simulink model "propagator"  (R2019b)
settings: Solver=VariableStepAuto  StartTime=0.0  StopTime=10.0  RelTol=1e-3
model workspace (MAT data in the model file):
  X0 = 1
  mi = 1
settings Model: Creator=antoniogenova  LastModifiedBy=antoniogenova

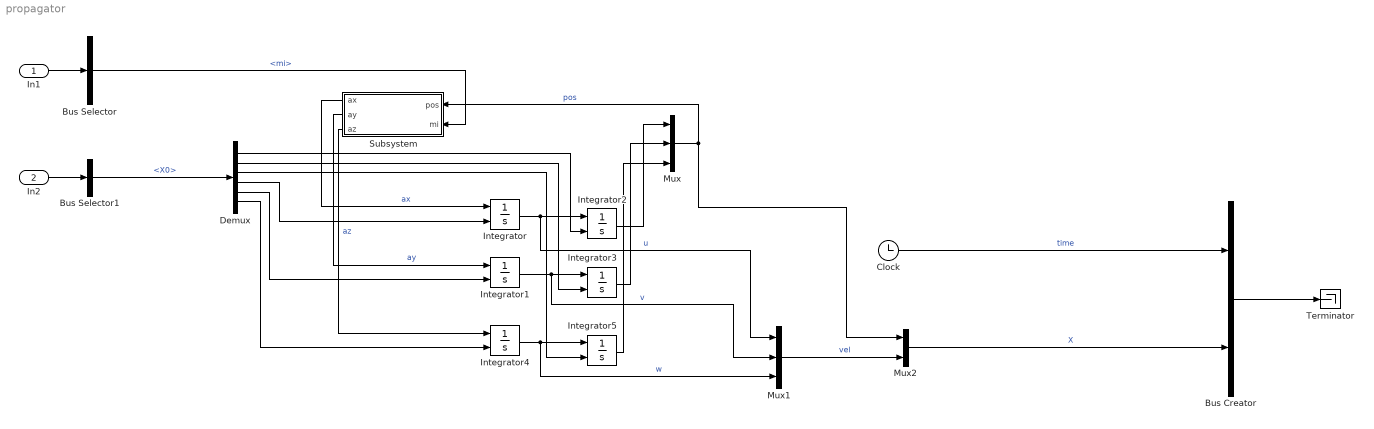
== system propagator ==
  In1 : Inport  OutDataTypeStr=Bus: ParBody_Bus
  In2 : Inport  Port=2  OutDataTypeStr=Bus: ParEphemerides_Bus
  Bus Creator : BusCreator  Inputs=2
  Bus Selector : BusSelector  OutputSignals=mi
  Bus Selector1 : BusSelector  OutputSignals=X0
  Clock : Clock
  Demux : Demux  Outputs=6
  Integrator{,1..5} (6 alike) : Integrator  InitialConditionSource=external  ContinuousStateAttributes="\"\""
  Mux : Mux  Inputs=3
  Mux1 : Mux  Inputs=3
  Mux2 : Mux  Inputs=2
  Subsystem : Subsystem
  Terminator : Terminator
  wires:
  Subsystem/1(ax) -> Integrator/1  "ax"
  Bus Creator/1 -> Terminator/1
  Demux/5 -> Integrator1/2
  Mux/1 -> Mux2/1, Subsystem/1(pos)  "pos"
  Integrator1/1 -> Mux1/2, Integrator3/1  "v"
  Mux1/1 -> Mux2/2  "vel"
  Demux/2 -> Integrator3/2
  Demux/1 -> Integrator2/2
  Subsystem/2(ay) -> Integrator1/1  "ay"
  Integrator/1 -> Mux1/1, Integrator2/1  "u"
  Integrator2/1 -> Mux/1
  Demux/6 -> Integrator4/2
  Integrator5/1 -> Mux/3
  Mux2/1 -> Bus Creator/2  "X"
  Integrator4/1 -> Mux1/3, Integrator5/1  "w"
  Subsystem/3(az) -> Integrator4/1  "az"
  Clock/1 -> Bus Creator/1  "time"
  Demux/4 -> Integrator/2
  Integrator3/1 -> Mux/2
  Demux/3 -> Integrator5/2
  In2/1 -> Bus Selector1/1
  In1/1 -> Bus Selector/1
  Bus Selector/1 -> Subsystem/2(mi)  "<mi>"
  Bus Selector1/1 -> Demux/1  "<X0>"

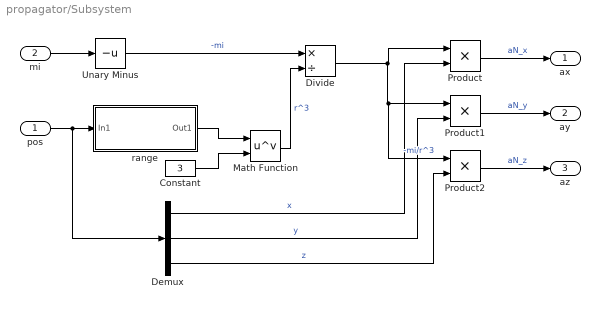
== system propagator/Subsystem ==
  pos : Inport
  mi : Inport  Port=2
  Constant : Constant  Value=3
  Demux : Demux  Outputs=3
  Divide : Product  Inputs=*/
  Math Function : Math  Operator=pow  SignedPower=off  SaturateOnIntegerOverflow=on
  Product : Product
  Product1 : Product
  Product2 : Product
  Unary Minus : UnaryMinus
  range : Subsystem
  ax : Outport
  ay : Outport  Port=2
  az : Outport  Port=3
  wires:
  pos/1 -> Demux/1, range/1(In1)
  mi/1 -> Unary Minus/1
  Unary Minus/1 -> Divide/1  "-mi"
  Constant/1 -> Math Function/2
  range/1(Out1) -> Math Function/1
  Math Function/1 -> Divide/2  "r^3"
  Divide/1 -> Product2/1, Product1/1, Product/1  "-mi/r^3"
  Demux/1 -> Product/2  "x"
  Demux/2 -> Product1/2  "y"
  Demux/3 -> Product2/2  "z"
  Product/1 -> ax/1  "aN_x"
  Product1/1 -> ay/1  "aN_y"
  Product2/1 -> az/1  "aN_z"

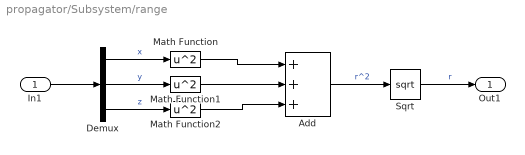
== system propagator/Subsystem/range ==
  In1 : Inport
  Add : Sum  Inputs=+++
  Demux : Demux  Outputs=3
  Math Function : Math  Operator=square  SignedPower=off  SaturateOnIntegerOverflow=on
  Math Function1 : Math  Operator=square  SignedPower=off  SaturateOnIntegerOverflow=on
  Math Function2 : Math  Operator=square  SignedPower=off  SaturateOnIntegerOverflow=on
  Sqrt : Sqrt  SaturateOnIntegerOverflow=on
  Out1 : Outport
  wires:
  In1/1 -> Demux/1
  Demux/1 -> Math Function/1  "x"
  Demux/2 -> Math Function1/1  "y"
  Demux/3 -> Math Function2/1  "z"
  Math Function/1 -> Add/1
  Math Function1/1 -> Add/2
  Math Function2/1 -> Add/3
  Add/1 -> Sqrt/1  "r^2"
  Sqrt/1 -> Out1/1  "r"
